simulink model "mljgz"  (R2022a)
settings: Solver=VariableStepAuto  StartTime=0.0  StopTime=50  RelTol=1e-3
values from neighbouring files (symbols this model uses):
  cx = [0 0.1 0.2 0.3 0.4 0.5 0.6 0.7 0.8 0.9 1 1.1 ... (1201 elements, 1x1201)]    [cx1.mat]
  cy = [0.00198252139388 0.00202092823424 0.00206007872329 0.00209998724464 0.0021406684595 0.00218213731203 0.0022244090348 0.00226749915428 0.00231142349654 0.00235619819297 0.00240183968615 0.00244836473584 ... (1201 elements, 1x1201)]    [cy1.mat]
undefined symbols (not defined in the file or in its folder): r_k, r_yaw
libraries: Solver_SF x1, simulink x1, slpidlib x1
settings Model: Creator=wenju  LastModifiedBy=wenju

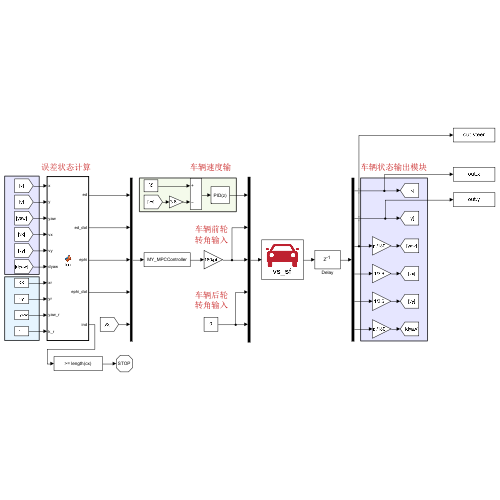
[thumbnail: Simulink's stored preview of the top-level diagram]
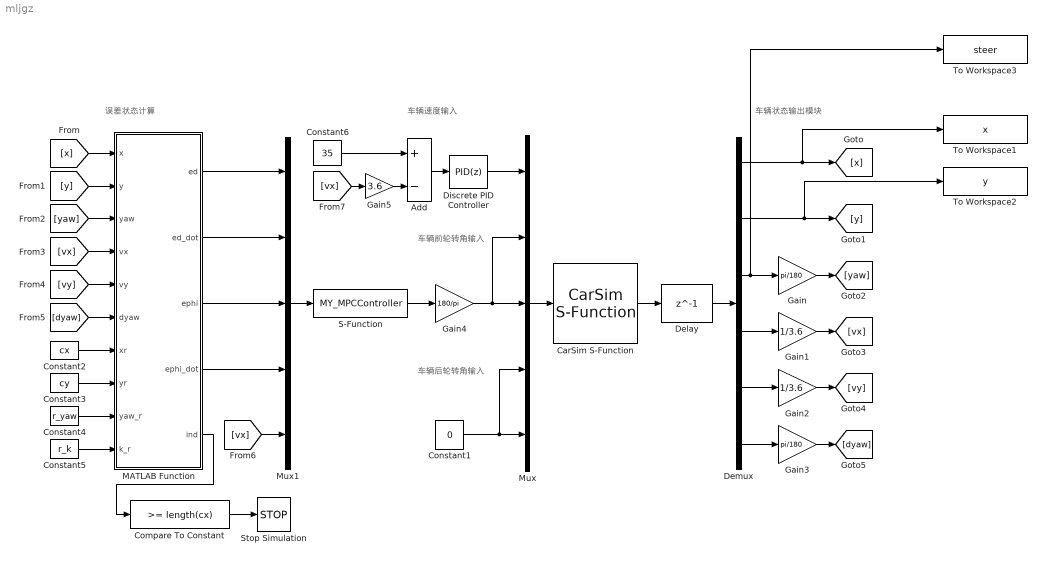
== system mljgz ==
  note: 误差状态计算
  note: 车辆状态输出模块
  note: 车辆速度输入
  note: 车辆后轮转角输入
  note: 车辆前轮转角输入
  Add : Sum  Inputs=+-
  CarSim S-Function : Solver_SF/CarSim S-Function  Priority=1  SIMFILE=simfile.sim  Run_RTs=off  vs_state_ind=Run  StopMode_ind=Vehicle Model
  Compare To Constant : simulink/Logic and Bit Operations/Compare To Constant  relop=>=  const=length(cx)  OutDataTypeStr=boolean
  Constant1 : Constant  Value=0
  Constant2 : Constant  Value=cx
  Constant3 : Constant  Value=cy
  Constant4 : Constant  Value=r_yaw
  Constant5 : Constant  Value=r_k
  Constant6 : Constant  Value=35
  Delay : Delay  DelayLength=1  InitialCondition=0  UseCircularBuffer=on
  Demux : Demux  Outputs=6
  Discrete PID Controller : slpidlib/PID Controller  Controller=PID  Form=Parallel  TimeDomain=Discrete-time  UseExternalTs=off  SampleTime=-1  IntegratorMethod=Forward Euler  FilterMethod=Forward Euler  ControllerParametersSource=internal  P=0.8  I=0.6  UseKiTs=off  D=0.2  N=100  UseFilter=off  TunerSelectOption=Transfer Function Based (PID Tuner App)  InitialConditionSource=internal  InitialConditionForIntegrator=0  InitialConditionForFilter=0  DifferentiatorICPrevScaledInput=0  ExternalReset=none  TrackingMode=off  Kt=1  LimitOutput=off  SatLimitsSource=internal  UpperSaturationLimit=inf  LowerSaturationLimit=-inf  LinearizeAsGain=off  AntiWindupMode=none  Kb=1  POutMin=[]  POutMax=[]  IOutMin=[]  IOutMax=[]  DOutMin=[]  DOutMax=[]  NOutMin=[]  NOutMax=[]  SumOutMin=[]  SumOutMax=[]  SaturationOutMin=[]  SaturationOutMax=[]  PParamMin=[]  PParamMax=[]  IParamMin=[]  IParamMax=[]  DParamMin=[]  DParamMax=[]  NParamMin=[]  NParamMax=[]  KbParamMin=[]  KbParamMax=[]  KtParamMin=[]  KtParamMax=[]  KbOutMin=[]  KbOutMax=[]  KtOutMin=[]  KtOutMax=[]  IntegratorOutMin=[]  IntegratorOutMax=[]  FilterOutMin=[]  FilterOutMax=[]  SumI1OutMin=[]  SumI1OutMax=[]  SumI2OutMin=[]  SumI2OutMax=[]  SumI3OutMin=[]  SumI3OutMax=[]  SumI4OutMin=[]  SumI4OutMax=[]  SumDOutMin=[]  SumDOutMax=[]  DifferentiatorOutMin=[]  DifferentiatorOutMax=[]  FilterDiffOutCoefMin=[]  FilterDiffOutCoefMax=[]  ReciprocalOutMin=[]  ReciprocalOutMax=[]  SumDenOutMin=[]  SumDenOutMax=[]  SumNumOutMin=[]  SumNumOutMax=[]  DivideOutMin=[]  DivideOutMax=[]  UdiffTsProdOutMin=[]  UdiffTsProdOutMax=[]  NTsProdOutMin=[]  NTsProdOutMax=[]  UintegralTsProdOutMin=[]  UintegralTsProdOutMax=[]  UngainTsProdOutMin=[]  UngainTsProdOutMax=[]  IntegratorContinuousStateAttributes=''  IntegratorStateMustResolveToSignalObject=off  IntegratorRTWStateStorageClass=Auto  FilterContinuousStateAttributes=''  FilterStateMustResolveToSignalObject=off  FilterRTWStateStorageClass=Auto  ParallelPVariant=InternalParameters  IdealPVariant=Disabled  IVariant=InternalParameters  DVariant=InternalParameters  IntegratorVariant=Discrete  SatVariant=Disabled  AWVariant=Passthrough  PCopyVariant=Disabled  TRVariant=Disabled  FdbkBlocksVariant=Forward  IdealPFdbkVariant=Disabled  SatFdbkVariant=Disabled  DerivativeFilterVariant=Differentiator  NVariant=Passthrough  NCopyVariant=Disabled_SignalSpec  FilterICVariant=InternalICsDifferentiator  IntegratorICVariant=InternalICs  ExternalResetVariant=Disabled  TRSumVariant=Passthrough  SumFdbkVariant=Disabled  SumVariant=Sum_PID  TsampFilterVariant=InternalTs  TsampNgainVariant=Passthrough  TsampIntegralVariant=Passthrough  ExternalSaturationOutDataTypeStr=Inherit: Same as second input  aMode=0
  Gain : Gain  Gain=pi/180
  Gain1 : Gain  Gain=1/3.6
  Gain2 : Gain  Gain=1/3.6
  Gain3 : Gain  Gain=pi/180
  Gain4 : Gain  Gain=180/pi
  Gain5 : Gain  Gain=3.6
  MATLAB Function : MATLAB Function  TreatAsAtomicUnit=on
  Mux : Mux  Inputs=5
  Mux1 : Mux  Inputs=5
  S-Function : S-Function  FunctionName=MY_MPCController  SFunctionDeploymentMode=off  EnableBusSupport=off
  Stop Simulation : Stop
  To Workspace1 : ToWorkspace  VariableName=x  SaveFormat=Timeseries  SampleTime=0.05
  To Workspace2 : ToWorkspace  VariableName=y  SaveFormat=Timeseries  SampleTime=0.05
  To Workspace3 : ToWorkspace  VariableName=steer  SaveFormat=Timeseries  SampleTime=0.05
  wires:
  CarSim S-Function/1 -> Delay/1
  Delay/1 -> Demux/1
  Demux/1 -> To Workspace1/1, [x]
  Demux/2 -> To Workspace2/1, [y]
  Demux/3 -> To Workspace3/1, Gain/1
  Gain/1 -> [yaw]
  Demux/4 -> Gain1/1
  Gain1/1 -> [vx]
  Demux/5 -> Gain2/1
  Gain2/1 -> [vy]
  Demux/6 -> Gain3/1
  Gain3/1 -> [dyaw]
  Mux/1 -> CarSim S-Function/1
  Constant1/1 -> Mux/4, Mux/5
  [x] -> MATLAB Function/1(x)
  [y] -> MATLAB Function/2(y)
  [yaw] -> MATLAB Function/3(yaw)
  [vx] -> MATLAB Function/4(vx)
  [vy] -> MATLAB Function/5(vy)
  [dyaw] -> MATLAB Function/6(dyaw)
  Constant2/1 -> MATLAB Function/7(xr)
  Constant3/1 -> MATLAB Function/8(yr)
  Constant4/1 -> MATLAB Function/9(yaw_r)
  Constant5/1 -> MATLAB Function/10(k_r)
  MATLAB Function/1(ed) -> Mux1/1
  MATLAB Function/2(ed_dot) -> Mux1/2
  MATLAB Function/3(ephi) -> Mux1/3
  MATLAB Function/4(ephi_dot) -> Mux1/4
  Mux1/1 -> S-Function/1
  S-Function/1 -> Gain4/1
  [vx] -> Mux1/5
  Compare To Constant/1 -> Stop Simulation/1
  MATLAB Function/5(ind) -> Compare To Constant/1
  Add/1 -> Discrete PID Controller/1
  Constant6/1 -> Add/1
  [vx] -> Gain5/1
  Gain5/1 -> Add/2
  Discrete PID Controller/1 -> Mux/1
  Gain4/1 -> Mux/2, Mux/3

== matlab function mljgz/MATLAB Function ==
  data: x input; ed output; y input; yaw input; vx input; vy input; dyaw input; xr input; yr input; yaw_r input; k_r input; ed_dot output; ephi output; ephi_dot output; ind output
function [ed,ed_dot,ephi,ephi_dot,ind] = fcn(x,y,yaw, vx,vy,dyaw,xr,yr,yaw_r,k_r)
%1.寻找匹配点（车辆离期望路径最近的点）   
    n=length(xr);
    d_min=(x-xr(1))^2+(y-yr(1))^2;
    min=1;
    for i=1:n
        d=(x-xr(i))^2+(y-yr(i))^2;
        if d<d_min
            d_min=d;
            min=i;
        end
    end
    ind=min;
%2.计算4个误差状态[ed,d_ed,eyaw,d_eyaw]
    tor=[cos(yaw_r(ind));sin(yaw_r(ind))];
    nor=[-sin(yaw_r(ind));cos(yaw_r(ind))];
    d_err=[x-xr(ind);y-yr(ind)];

    ed=nor'*d_err;
%     es=tor'*d_err; 
    projection_point_thetar=yaw_r(ind); %百度apollo

    ed_dot=vy*cos(yaw-projection_point_thetar)+vx*sin(yaw-projection_point_thetar);
    ephi=sin(yaw-projection_point_thetar);
    s_dot=vx*cos(yaw-projection_point_thetar)-vy*sin(yaw-projection_point_thetar);
    s_dot=s_dot/(1-k_r(ind)*ed);
    ephi_dot=dyaw-k_r(ind)*s_dot;

end
